simulink model "simrect"  (R2015a)
settings: Solver=ode45  StartTime=0.0  StopTime=1000  RelTol=1e-3
libraries: powerlib x6
settings Model: Creator=Kelvin Gakuo  LastModifiedBy=Kelvin Gakuo

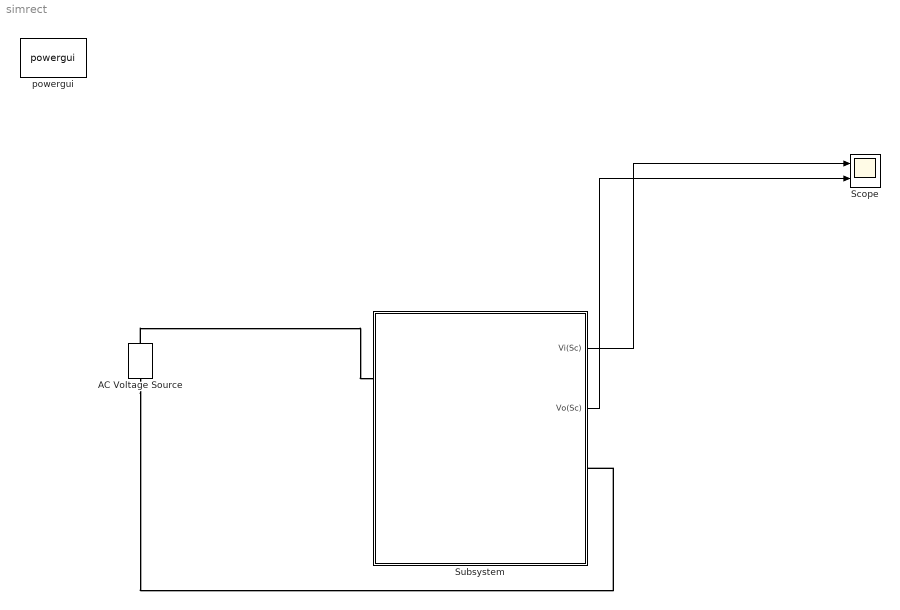
== system simrect ==
  AC Voltage Source : powerlib/Electrical Sources/AC Voltage Source  Amplitude=40.84  Phase=0  Frequency=50  SampleTime=0  Measurements=None
  Scope : Scope  NumInputPorts=2
      settings: TimeRange=0.1  YMin=-45~-2.5  YMax=45~42.5
  Subsystem : Subsystem
  powergui : powerlib/powergui  Priority=1  SimulationMode=Continuous  SolverType=Tustin/Backward Euler (TBE)  SampleTime=50e-6  frequency=60  SPID=on  DisableSnubberDevices=off  DisableRonSwitches=off  DisableVfSwitches=off  SwTol=0  DisplayEquations=off  Interpol=off  methode=off  Ts=100  FunctionMessages=off  echomessages=off  HookPort=off  EnableUseOfTLC=off  x0status=blocks  frequencyindice=0  Pbase=100e6  ErrMax=1e-4  Iterations=50  UnitsV=kV  UnitsW=MW  buscounter=0  RestoreLinks=warning  ResistiveCurrentMeasurement=off  Frange=[0:2:500]  Ylog=off  Xlog=on  ShowGrid=off  save=off  variable=ZData  structure=0  ZoomFFT=off  StartTime=0.0  cycles=1  DisplayStyle=1  fundamental=60  FreqAxis=off  MaxFrequency=1000  frequencyindicesteady=1  RmsSteady=1  display=off
  wires:
  Subsystem/1(Vi(Sc)) -> Scope/1
  Subsystem/2(Vo(Sc)) -> Scope/2
  connections:
  AC Voltage Source/RConn1 -- Subsystem/LConn1
  AC Voltage Source/LConn1 -- Subsystem/RConn1

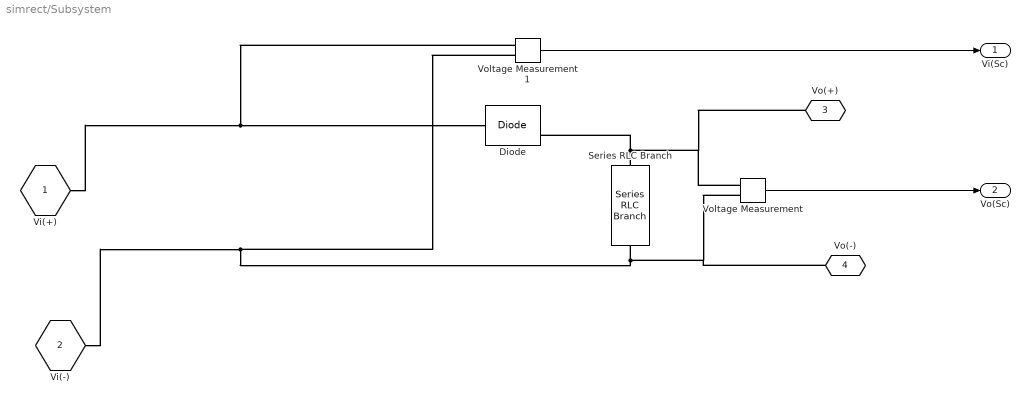
== system simrect/Subsystem ==
  Diode : powerlib/Power Electronics/Diode  Ron=0.001  Lon=0  Vf=0.8  IC=0  UseSnubber=off  Rs=500  Cs=250e-9  Measurements=on
  Series RLC Branch : powerlib/Elements/Series RLC Branch  LConnTagsString=__new0  RConnTagsString=__new0  BranchType=R  Resistance=40.81  Inductance=1e-3  SetiL0=off  InitialCurrent=0  Capacitance=1e-6  Setx0=off  InitialVoltage=0  Measurements=None
  Voltage Measurement : powerlib/Measurements/Voltage Measurement  PhasorSimulation=off  OutputType=Complex  PSBequivalent=0
  Voltage Measurement1 : powerlib/Measurements/Voltage Measurement  PhasorSimulation=off  OutputType=Complex  PSBequivalent=0
  Vi(+) : PMIOPort  Port=1  Side=Left
  Vi(-) : PMIOPort  Port=2  Side=Right
  Vo(+) : PMIOPort  Port=3  Side=Left
  Vo(-) : PMIOPort  Port=4  Side=Right
  Vi(Sc) : Outport
  Vo(Sc) : Outport  Port=2
  wires:
  Voltage Measurement/1 -> Vo(Sc)/1
  Voltage Measurement1/1 -> Vi(Sc)/1
  connections:
  Voltage Measurement1/LConn1 -- Vi(+)/RConn1 -- Diode/LConn1
  Voltage Measurement1/LConn2 -- Vi(-)/RConn1 -- Voltage Measurement/LConn2 -- Vo(-)/RConn1 -- Series RLC Branch/RConn1
  Series RLC Branch/LConn1 -- Voltage Measurement/LConn1 -- Vo(+)/RConn1 -- Diode/RConn1
